simulink model "WorkerProductivity"  (R2024b)
settings: Solver=FixedStepAuto  StartTime=0.0  StopTime=10.0  FixedStep=0.01  RelTol=1e-3
settings Model: Creator=max  LastModifiedBy=max

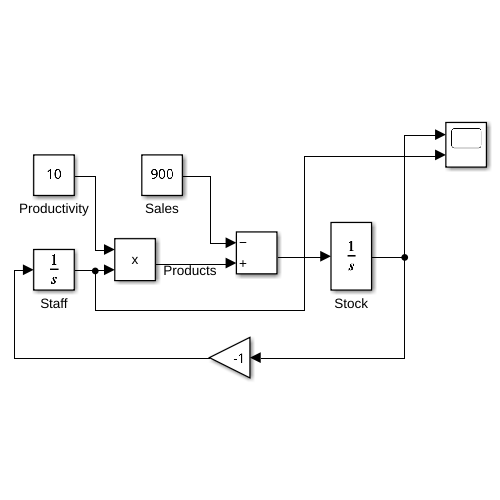
[thumbnail: Simulink's stored preview of the top-level diagram]
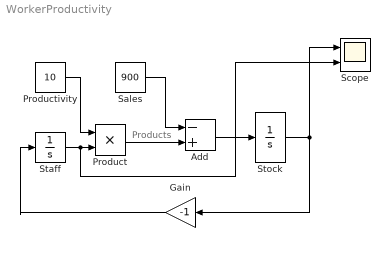
== system WorkerProductivity ==
  note: Products
  Add : Sum  Inputs=-+
  Gain : Gain  Gain=-1
  Product : Product
  Productivity : Constant  Value=10
  Sales : Constant  Value=900
  Scope : Scope  NumInputPorts=2
  Staff : Integrator
  Stock : Integrator
  wires:
  Stock/1 -> Scope/1, Gain/1
  Add/1 -> Stock/1
  Sales/1 -> Add/1
  Staff/1 -> Scope/2, Product/2
  Product/1 -> Add/2
  Productivity/1 -> Product/1
  Gain/1 -> Staff/1
